simulink model "quadrotor_model50"  (R2021a)
settings: Solver=VariableStepAuto  StartTime=0.0  StopTime=40  RelTol=1e-1
values from neighbouring files (symbols this model uses):
  X = [X realx(index)]    [Plot_drone_3D.m]    (also in Plot_drone_3D_sub.m)
  Y = [Y realy(index)]    [Plot_drone_3D.m]    (also in Plot_drone_3D_sub.m)
  Z = [Z realz(index)]    [Plot_drone_3D.m]    (also in Plot_drone_3D_sub.m)
undefined symbols (not defined in the file or in its folder): Discrete, Time
libraries: sm_lib x6, sharedTrackingLibrary x4, sharedtransform x3, vrlib x2, aerolibutil x2, nesl_utility x1, dspmtrx3 x1, ctrlSharedLib x1
(part 1 of 2)
settings Model: EnablePacing=on  PacingRate=50  Creator=amejiyopakapak  LastModifiedBy=user
settings DataIOCC: ReturnWorkspaceOutputs=off
settings DebuggingCC: UnderSpecifiedDimensionMsg=warning

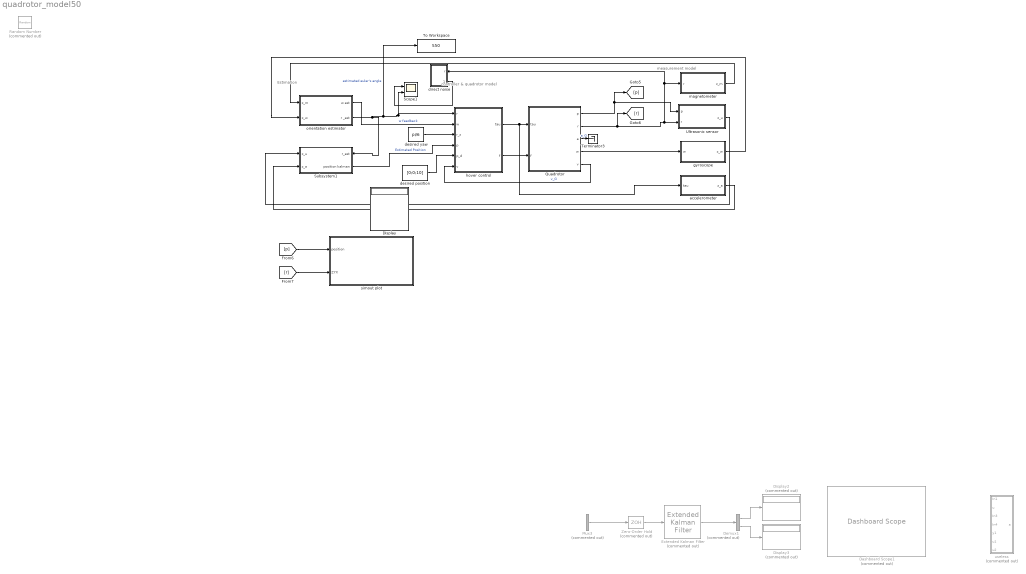
== system quadrotor_model50 ==
  note: Estimation
  note: measurement model
  note: controller & quadrotor model
  Dashboard Scope1 : DashboardScope  Commented=on
  Demux1 : Demux  Commented=on  Outputs=2
  Display : Display
  Display2 : Display  Commented=on
  Display3 : Display  Commented=on
  Extended Kalman Filter : sharedTrackingLibrary/Extended Kalman Filter  Commented=on  StateTransitionFcn=state  HasStateTransitionJacobianFcn=on  HasAdditiveProcessNoise=Nonadditive  ProcessNoise=[[1;1;1];[1;1;1]]  HasTimeVaryingProcessNoise=off  HasStateTransitionFcnExtraArgument=0  InitialState=[[0;0;0];[0;0;0]]  InitialStateCovariance=[[1;1;1];[1;1;1]]  MeasurementFcn1=measurement  HasMeasurementJacobianFcn1=off  HasMeasurementEnablePort1=off  HasAdditiveMeasurementNoise1=Additive  MeasurementNoise1=[[1;1;1];[1;1;1]]  HasTimeVaryingMeasurementNoise1=off  HasMeasurementFcnExtraArgument1=0  MeasurementFcn2=myMeasurementFcn  HasMeasurementJacobianFcn2=off  HasMeasurementEnablePort2=off  HasAdditiveMeasurementNoise2=Additive  MeasurementNoise2=1  HasTimeVaryingMeasurementNoise2=off  HasMeasurementFcnExtraArgument2=0  MeasurementFcn3=myMeasurementFcn  HasMeasurementJacobianFcn3=off  HasMeasurementEnablePort3=off  HasAdditiveMeasurementNoise3=Additive  MeasurementNoise3=1  HasTimeVaryingMeasurementNoise3=off  HasMeasurementFcnExtraArgument3=0  MeasurementFcn4=myMeasurementFcn  HasMeasurementJacobianFcn4=off  HasMeasurementEnablePort4=off  HasAdditiveMeasurementNoise4=Additive  MeasurementNoise4=1  HasTimeVaryingMeasurementNoise4=off  HasMeasurementFcnExtraArgument4=0  MeasurementFcn5=myMeasurementFcn  HasMeasurementJacobianFcn5=off  HasMeasurementEnablePort5=off  HasAdditiveMeasurementNoise5=Additive  MeasurementNoise5=1  HasTimeVaryingMeasurementNoise5=off  HasMeasurementFcnExtraArgument5=0  EnableMultirate=off  StateTransitionFcnSampleTime=1  MeasurementFcn1SampleTime=1  MeasurementFcn2SampleTime=1  MeasurementFcn3SampleTime=1  MeasurementFcn4SampleTime=1  MeasurementFcn5SampleTime=1  UseCurrentEstimator=on  OutputStateCovariance=off  DataType=double  SampleTime=0.01  NumberOfMeasurements=1
      settings: SourceProductBaseCode=CT,DR,TF,ID,LP,NV,AR,RO,RR,UV,VE
  Mux3 : Mux  Commented=on  Inputs=2
  Quadrotor : Subsystem
  Random Number : RandomNumber  Commented=on  SampleTime=0.1
  Scope1 : Scope  NumInputPorts=2
  Subsystem1 : Subsystem
      settings: PortSchema="{\"entries\":[{\"content\":{\"sides\":[{\"content\":{\"connectorIds\":[\"In1\",\"In2\"]},\"type\":\"ConnectorPlacement.EquallySpacedRectSide\",\"uuid\":\"ff0e47d5-67a6-410d-af15-00f9184d5f56\"},{\"content\":{\"connectorIds\":[\"In3\",\"Out1\"],\"side\":\"RIGHT\"},\"type\":\"ConnectorPlacement.EquallySpacedRectSide\",\"uuid\":\"3604025b-9f7e-46ce-b48f-09d2018bc808\"},{\"content\":{\"connectorIds\":[],\"side\":\"TOP\"},\"type\":\"ConnectorPlacement.EquallySpacedRectSide\",\"uuid\":\"c6ccdc8d-b714-489c-bc8f-943c64a4c150\"}]},\"type\":\"ConnectorPlacement.EquallySpacedConnector\",\"uuid\":\"6526fc3b-b978-451b-84c0-583e32a0b9e3\"}],\"packageUris\":[\"http://schema.mathworks.com/mf0/Connector/R2020b\"],\"version\":\"1.0\"}"
  Terminator3 : Terminator
  To Workspace : ToWorkspace  VariableName=S50  SaveFormat=Timeseries  SampleTime=1/50
  Ultrasonic sensor : Subsystem
  Zero-Order Hold : ZeroOrderHold  Commented=on  SampleTime=0.01
  accelerometer : Subsystem
  desired position : Constant  Value=[0;0;10]
  desired yaw : Constant  Value=pi/6
  direct noise : Subsystem
      settings: PortSchema="{\"entries\":[{\"content\":{\"sides\":[{\"content\":{\"connectorIds\":[]},\"type\":\"ConnectorPlacement.EquallySpacedRectSide\",\"uuid\":\"c51df378-8ff8-4d17-a243-2bd48f2a1343\"},{\"content\":{\"connectorIds\":[\"In1\",\"Out1\"],\"side\":\"RIGHT\"},\"type\":\"ConnectorPlacement.EquallySpacedRectSide\",\"uuid\":\"e335f112-6ed8-4a5c-b285-a63f6c692f38\"},{\"content\":{\"connectorIds\":[],\"side\":\"TOP\"},\"type\":\"ConnectorPlacement.EquallySpacedRectSide\",\"uuid\":\"f87c7cdc-99df-462c-be44-1c188cc81712\"}]},\"type\":\"ConnectorPlacement.EquallySpacedConnector\",\"uuid\":\"5aacd153-2f27-4b85-80cd-18cd67604917\"}],\"packageUris\":[\"http://schema.mathworks.com/mf0/Connector/R2020b\"],\"version\":\"1.0\"}"
  gyroscope : Subsystem
  hover control : Subsystem  mask{mass=1}
  magnetometer : Subsystem
      settings: PortSchema="{\"entries\":[{\"content\":{\"sides\":[{\"content\":{\"connectorIds\":[\"Out1\"]},\"type\":\"ConnectorPlacement.EquallySpacedRectSide\",\"uuid\":\"28b5311d-12b5-46a9-9a41-026d4bdaef13\"},{\"content\":{\"connectorIds\":[\"In1\"],\"side\":\"RIGHT\"},\"type\":\"ConnectorPlacement.EquallySpacedRectSide\",\"uuid\":\"3c807059-2a43-4a59-b0f2-7f82e794ec70\"},{\"content\":{\"connectorIds\":[],\"side\":\"TOP\"},\"type\":\"ConnectorPlacement.EquallySpacedRectSide\",\"uuid\":\"12203a37-ceaf-447f-ac57-ca6e6fe841d3\"}]},\"type\":\"ConnectorPlacement.EquallySpacedConnector\",\"uuid\":\"1f119634-8b2a-4a6d-a5af-b856cc81d6c9\"}],\"packageUris\":[\"http://schema.mathworks.com/mf0/Connector/R2020b\"],\"version\":\"1.0\"}"
  orientation estimator : Subsystem
  simout plot : Subsystem
  useless : Subsystem  Commented=on
  wires:
  desired yaw/1 -> hover control/3(r_z)
  Quadrotor/5(v) -> hover control/6(v)  "v_G"
  hover control/1(tau) -> accelerometer/1(tau), Quadrotor/1(tau)
  desired position/1 -> hover control/5(p_d)
  hover control/2(f) -> Quadrotor/2(f)
  Quadrotor/1(p) -> Ultrasonic sensor/1(p), [p]
  Mux3/1 -> Zero-Order Hold/1
  Extended Kalman Filter/1 -> Demux1/1
  Demux1/1 -> Display2/1
  Demux1/2 -> Display3/1
  Zero-Order Hold/1 -> Extended Kalman Filter/1
  orientation estimator/1(w est) -> hover control/2(w)  "w feedback"
  Quadrotor/4(w) -> gyroscope/1(w)
  Quadrotor/3(a) -> Terminator3/1  "a_G"
  magnetometer/1(z_m) -> orientation estimator/1(z_m)
  gyroscope/1(z_w) -> orientation estimator/2(z_w)
  accelerometer/1(z_a) -> Subsystem1/2(z_a)
  orientation estimator/2(r _est) -> Subsystem1/3(r_est), To Workspace/1, Scope1/2, hover control/1(r)  "estimated euler's angle"
  [p] -> simout plot/1(position)
  [r] -> simout plot/2(ZYX)
  Ultrasonic sensor/1(z_u) -> Subsystem1/1(z_u)
  Subsystem1/1(position kalman) -> hover control/4(p)  "Estimated Position"
  Quadrotor/2(r) -> direct noise/1(r), magnetometer/1(r), Ultrasonic sensor/2(r), [r]
  direct noise/1(ZYX) -> Scope1/1

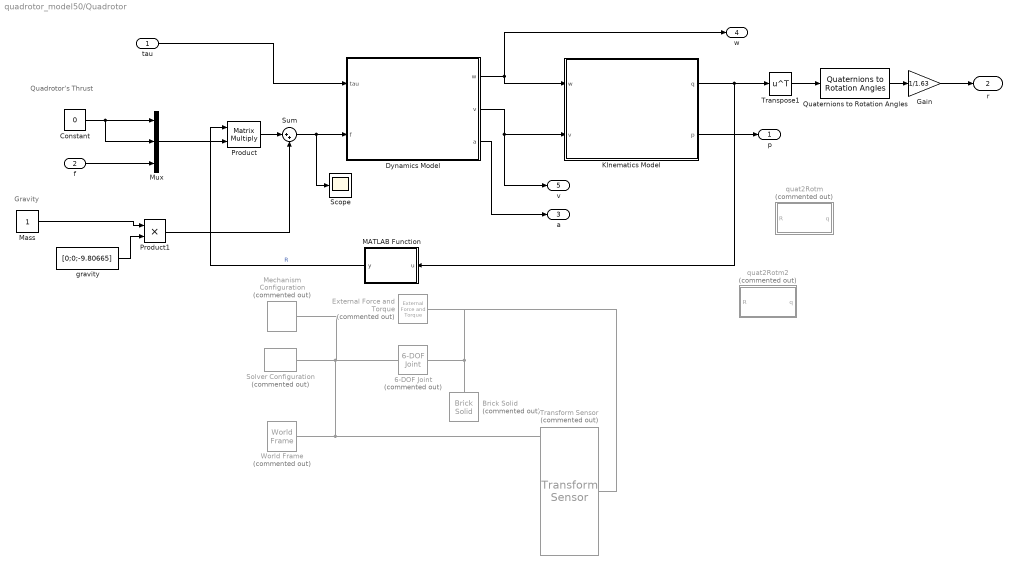
== system quadrotor_model50/Quadrotor ==
  note: Quadrotor's Thrust
  note: Gravity
  tau : Inport  SampleTime=1/50
  f : Inport  Port=2  SampleTime=1/50
  6-DOF Joint : sm_lib/Joints/6-DOF Joint  Commented=on  JointMode=Normal  SenseConstraintForce=off  SenseConstraintForceX=off  SenseConstraintForceY=off  SenseConstraintForceZ=off  SenseConstraintTorque=off  SenseConstraintTorqueX=off  SenseConstraintTorqueY=off  SenseConstraintTorqueZ=off  SenseTotalForce=off  SenseTotalForceX=off  SenseTotalForceY=off  SenseTotalForceZ=off  SenseTotalTorque=off  SenseTotalTorqueX=off  SenseTotalTorqueY=off  SenseTotalTorqueZ=off  CompositeWrenchDir=FollowerOnBase  CompositeWrenchFrame=BaseFrame  PxEquilibriumPosition=0  PxEquilibriumPositionUnits=m  PxSpringStiffness=0  PxSpringStiffnessUnits=N/m  PxDampingCoefficient=0  PxDampingCoefficientUnits=N/(m/s)  PxTorqueActuationMode=NoTorque  PxMotionActuationMode=ComputedMotion  PxSensePosition=off  PxSenseVelocity=off  PxSenseAcceleration=off  PxSenseTorqueForce=off  PxSenseLowerLimitTorqueForce=off  PxSenseUpperLimitTorqueForce=off  PxLowerLimitSpecify=off  PxLowerLimitBound=-1  PxLowerLimitBoundUnits=m  PxLowerLimitStiffness=1e6  PxLowerLimitStiffnessUnits=N/m  PxLowerLimitDamping=1e3  PxLowerLimitDampingUnits=N/(m/s)  PxLowerLimitTransitionRegionWidth=1e-4  PxLowerLimitTransitionRegionWidthUnits=m  PxUpperLimitSpecify=off  PxUpperLimitBound=1  PxUpperLimitBoundUnits=m  PxUpperLimitStiffness=1e6  PxUpperLimitStiffnessUnits=N/m  PxUpperLimitDamping=1e3  PxUpperLimitDampingUnits=N/(m/s)  PxUpperLimitTransitionRegionWidth=1e-4  PxUpperLimitTransitionRegionWidthUnits=m  PxPositionTargetSpecify=off  PxPositionTargetPriority=High  PxPositionTargetValue=0  PxPositionTargetValueUnits=m  PxVelocityTargetSpecify=off  PxVelocityTargetPriority=High  PxVelocityTargetValue=0  PxVelocityTargetValueUnits=m/s  PyEquilibriumPosition=0  PyEquilibriumPositionUnits=m  PySpringStiffness=0  PySpringStiffnessUnits=N/m  PyDampingCoefficient=0  PyDampingCoefficientUnits=N/(m/s)  PyTorqueActuationMode=NoTorque  PyMotionActuationMode=ComputedMotion  PySensePosition=off  PySenseVelocity=off  PySenseAcceleration=off  PySenseTorqueForce=off  PySenseLowerLimitTorqueForce=off  PySenseUpperLimitTorqueForce=off  PyLowerLimitSpecify=off  PyLowerLimitBound=-1  PyLowerLimitBoundUnits=m  PyLowerLimitStiffness=1e6  PyLowerLimitStiffnessUnits=N/m  PyLowerLimitDamping=1e3  PyLowerLimitDampingUnits=N/(m/s)  PyLowerLimitTransitionRegionWidth=1e-4  PyLowerLimitTransitionRegionWidthUnits=m  PyUpperLimitSpecify=off  PyUpperLimitBound=1  PyUpperLimitBoundUnits=m  PyUpperLimitStiffness=1e6  PyUpperLimitStiffnessUnits=N/m  PyUpperLimitDamping=1e3  PyUpperLimitDampingUnits=N/(m/s)  PyUpperLimitTransitionRegionWidth=1e-4  PyUpperLimitTransitionRegionWidthUnits=m  PyPositionTargetSpecify=off  PyPositionTargetPriority=High  PyPositionTargetValue=0  PyPositionTargetValueUnits=m  PyVelocityTargetSpecify=off  PyVelocityTargetPriority=High  PyVelocityTargetValue=0  PyVelocityTargetValueUnits=m/s  PzEquilibriumPosition=0  PzEquilibriumPositionUnits=m  PzSpringStiffness=0  PzSpringStiffnessUnits=N/m  PzDampingCoefficient=0  PzDampingCoefficientUnits=N/(m/s)  PzTorqueActuationMode=NoTorque  PzMotionActuationMode=ComputedMotion  PzSensePosition=off  PzSenseVelocity=off  PzSenseAcceleration=off  PzSenseTorqueForce=off  PzSenseLowerLimitTorqueForce=off  PzSenseUpperLimitTorqueForce=off  PzLowerLimitSpecify=off  PzLowerLimitBound=-1  PzLowerLimitBoundUnits=m  PzLowerLimitStiffness=1e6  PzLowerLimitStiffnessUnits=N/m  PzLowerLimitDamping=1e3  PzLowerLimitDampingUnits=N/(m/s)  PzLowerLimitTransitionRegionWidth=1e-4  PzLowerLimitTransitionRegionWidthUnits=m  PzUpperLimitSpecify=off  PzUpperLimitBound=1  PzUpperLimitBoundUnits=m  PzUpperLimitStiffness=1e6  PzUpperLimitStiffnessUnits=N/m  PzUpperLimitDamping=1e3  PzUpperLimitDampingUnits=N/(m/s)  PzUpperLimitTransitionRegionWidth=1e-4  PzUpperLimitTransitionRegionWidthUnits=m  PzPositionTargetSpecify=off  PzPositionTargetPriority=High  PzPositionTargetValue=0  PzPositionTargetValueUnits=m  PzVelocityTargetSpecify=off  PzVelocityTargetPriority=High  PzVelocityTargetValue=0  PzVelocityTargetValueUnits=m/s  SphDefPosRotationMethod=None  SphDefPosRotationAngleUnits=deg  SphDefPosRotationStandardAxis=+Z  SphDefPosRotationAngle=0.0  SphDefPosRotationArbitraryAxis=[0 0 1]  SphDefPosFollAlignAxisA=+X  SphDefPosBaseAlignAxisA=+Y  SphDefPosFollAlignAxisB=+Y  SphDefPosBaseAlignAxisB=+Z  SphDefPosRotationSequenceAxes=FollowerAxes  SphDefPosRotationSequence=XYX  SphDefPosRotationSequenceAngles=[0 0 0]  SphDefPosRotationSequenceAnglesUnits=deg  SphDefPosRotationMatrix=[1 0 0; 0 1 0; 0 0 1]  SphEqPosRotationMethod=None  SphEqPosRotationAngleUnits=deg  SphEqPosRotationStandardAxis=+Z  SphEqPosRotationAngle=0.0  SphEqPosRotationArbitraryAxis=[0 0 1]  SphEqPosFollAlignAxisA=+X  SphEqPosBaseAlignAxisA=+Y  SphEqPosFollAlignAxisB=+Y  SphEqPosBaseAlignAxisB=+Z  SphEqPosRotationSequenceAxes=FollowerAxes  SphEqPosRotationSequence=XYX  SphEqPosRotationSequenceAngles=[0 0 0]  SphEqPosRotationSequenceAnglesUnits=deg  SphEqPosRotationMatrix=[1 0 0; 0 1 0; 0 0 1]  SphSpringStiffness=0  SphSpringStiffnessUnits=N*m/deg  SphDampingCoefficient=0  SphDampingCoefficientUnits=N*m/(deg/s)  SphActuateTorqueX=off  SphActuateTorqueY=off  SphActuateTorqueZ=off  SphActuateTorque=off  SphTorqueActuationMode=NoTorque  SphMotionActuationMode=ComputedMotion  SphActuationFrame=BaseFrame  SphSensePosition=off  SphSenseVelocityX=off  SphSenseVelocityY=off  SphSenseVelocityZ=off  SphSenseVelocity=off  SphSenseAccelerationX=off  SphSenseAccelerationY=off  SphSenseAccelerationZ=off  SphSenseAcceleration=off  SphSenseTorqueX=off  SphSenseTorqueY=off  SphSenseTorqueZ=off  SphSenseTorqueForce=off  SphSenseLowerLimitTorqueMag=off  SphSenseUpperLimitTorqueMag=off  SphSensingFrame=BaseFrame  SphLowerLimitSpecify=off  SphLowerLimitBound=15  SphLowerLimitBoundUnits=deg  SphLowerLimitStiffness=1e4  SphLowerLimitStiffnessUnits=N*m/deg  SphLowerLimitDamping=10  SphLowerLimitDampingUnits=N*m/(deg/s)  SphLowerLimitTransitionRegionWidth=0.1  SphLowerLimitTransitionRegionWidthUnits=deg  SphUpperLimitSpecify=off  SphUpperLimitBound=45  SphUpperLimitBoundUnits=deg  SphUpperLimitStiffness=1e4  SphUpperLimitStiffnessUnits=N*m/deg  SphUpperLimitDamping=10  SphUpperLimitDampingUnits=N*m/(deg/s)  SphUpperLimitTransitionRegionWidth=0.1  SphUpperLimitTransitionRegionWidthUnits=deg  SphPositionTargetRotationMethod=None  SphPositionTargetRotationAngleUnits=deg  SphPositionTargetRotationStandardAxis=+Z  SphPositionTargetRotationAngle=0.0  SphPositionTargetRotationArbitraryAxis=[0 0 1]  SphPositionTargetFollAlignAxisA=+X  SphPositionTargetBaseAlignAxisA=+Y  SphPositionTargetFollAlignAxisB=+Y  SphPositionTargetBaseAlignAxisB=+Z  SphPositionTargetRotationSequenceAxes=FollowerAxes  SphPositionTargetRotationSequence=XYX  SphPositionTargetRotationSequenceAngles=[0 0 0]  SphPositionTargetRotationSequenceAnglesUnits=deg  SphPositionTargetRotationMatrix=[1 0 0; 0 1 0; 0 0 1]  SphPositionTargetSpecify=off  SphPositionTargetPriority=High  SphVelocityTargetValue=[0 0 0]  SphVelocityTargetValueUnits=deg/s  SphVelocityTargetSpecify=off  SphVelocityTargetPriority=High  SphVelocityTargetInFollowerFrame=on
  Brick Solid : sm_lib/Body Elements/Brick Solid  Commented=on  GraphicAmbientColor=[0.15 0.15 0.15 1.0]  BasedOnType=Density  BrickDimensions=[1 1 1]  BrickDimensionUnits=m  CenterOfMass=[0 0 0]  CenterOfMassUnits=m  GraphicDiffuseColor=[0.5 0.5 0.5]  Density=1000  DensityUnits=kg/m^3  DoExposeReferenceFrame=on  GraphicEmissiveColor=[0.0 0.0 0.0 1.0]  ExportEntireGeometry=off  SerializedFrames=<Frames/>  MarkerShape=Sphere  MarkerSize=10  GraphicType=FromGeometry  InertiaType=CalculateFromGeometry  Mass=1  MassUnits=kg  MomentsOfInertia=[1 1 1]  MomentsOfInertiaUnits=kg*m^2  GraphicOpacity=1.0  ProductsOfInertia=[0 0 0]  ProductsOfInertiaUnits=kg*m^2  GraphicShininess=75  GraphicSpecularColor=[0.5 0.5 0.5 1.0]  GraphicVisPropType=SimpleVisualProperties
  Constant : Constant  Value=0
  Dynamics Model : Subsystem  mask{I=[1 0 0 ; 0 1 0; 0 0 1], m=1, w_0=[0;0;0], v_0=[0;0;0]}
      mask prompts: I "Body Inertia Matrix"; m "Mass"; w_0 "Initial Angular Velocity"; v_0 "Initial Linear Velocity"
      mask DialogControl Container3 Prompt: Physical Parameters
      mask DialogControl Container4 Prompt: Initial States
      mask Display: disp('Dynamics Model')
  External Force and Torque : sm_lib/Forces and Torques/External Force and Torque  Commented=on  ForceResolutionFrame=AttachedFrame  EnableForceX=off  EnableForceY=off  EnableForceZ=off  EnableForce=on  TorqueResolutionFrame=AttachedFrame  EnableTorqueX=off  EnableTorqueY=off  EnableTorqueZ=off  EnableTorque=on
  Gain : Gain  Gain=1/1.63
  "KInematics Model " : Subsystem  mask{q_0=[1;0;0;0], p_0=[0;0;0]}
      mask prompts: q_0 "Initial Orienetation (in quaternion)"; p_0 "Initial Position"
      mask DialogControl Container3 Prompt: Initial States
      mask Display: disp('Kinematics Model')
  MATLAB Function : MATLAB Function  TreatAsAtomicUnit=on
  Mass : Constant
  Mechanism Configuration : sm_lib/Utilities/Mechanism Configuration  Commented=on  UniformGravity=Constant  GravityVector=[0 0 -9.80665]  GravityVectorUnits=m/s^2  GravityUnits=m/s^2  LinearizationDelta=0.001  JointModeTransitionNonlinearIterations=2
  Mux : Mux  Inputs=3
  Product : Product  Multiplication=Matrix(*)
  Product1 : Product
  Quaternions to Rotation Angles : sharedtransform/Quaternions to Rotation Angles  rotationOrder=ZYX  aMode=aMode
      settings: SourceProductBaseCode=AE,PW,DR,MT,UV,VE
  Scope : Scope
  Solver Configuration : nesl_utility/Solver Configuration  Commented=on  PhysicalDomain=network_engine_domain  SubClassName=solver  LeftPortType=input  RightPortType=generic  Tones=[]  Harmonics=[]  SimulateNoise=off  Profile=off  UseLocalSampling=off  EnableSwitchedLinearOptims=on  FrequencyDomain=off  UseCCode=off  RelTol=0.001  AbsTol=1e-06  MinStep=1e-09  ToWorkspace=off  RevertToSquareIcSolve=off  NumHomotopyIterations=100  PhasorMode=off  PhasorModeNumHarmonics=1  DoDC=off  ResidualTolerance=1e-09  UseLocalSolver=off  LocalSolverChoice=NE_BACKWARD_EULER_ADVANCER  LocalSolverSampleTime=0.001  DoFixedCost=off  MaxNonlinIter=3  MaxModeIter=2  ComputeImpulses=off  ImpulseIterations=2  LinearAlgebra=auto  EquationFormulation=NE_TIME_EF  DelaysMemoryBudget=1024  AutomaticFiltering=on  FilteringTimeConstant=0.001  PartitionStorageMethod=AS_NEEDED  PartitionMemoryBudget=1024  PartitionMethod=ROBUST
  Sum : Sum  Inputs=|++
  Transform Sensor : sm_lib/Frames and Transforms/Transform Sensor  Commented=on  MeasurementFrame=World  SenseAngle=off  SenseAxis=off  SenseAngle1=off  SenseAngle2=off  SenseAngle3=off  SenseQ=on  SenseR=off  SenseOmegaX=on  SenseOmegaY=on  SenseOmegaZ=on  SenseOmega1=off  SenseOmega2=off  SenseOmega3=off  SenseQDot=off  SenseRDot=off  SenseAlphaX=off  SenseAlphaY=off  SenseAlphaZ=off  SenseAlpha1=off  SenseAlpha2=off  SenseAlpha3=off  SenseQDDot=off  SenseRDDot=off  SenseX=on  SenseY=on  SenseZ=on  SenseRad=off  SenseAzim=off  SenseDist=off  SenseInc=off  SenseXDot=on  SenseYDot=on  SenseZDot=on  SenseRadDot=off  SenseAzimDot=off  SenseDistDot=off  SenseIncDot=off  SenseXDDot=off  SenseYDDot=off  SenseZDDot=off  SenseRadDDot=off  SenseAzimDDot=off  SenseDistDDot=off  SenseIncDDot=off
  Transpose1 : Math  Operator=transpose  SaturateOnIntegerOverflow=on
  World Frame : sm_lib/Frames and Transforms/World Frame  Commented=on
  gravity : Constant  Value=[0;0;-9.80665]
  quat2Rotm : Subsystem  Commented=on
      mask Display: disp('R(q)')
  quat2Rotm2 : Subsystem  Commented=on
      mask Display: disp('R(q)')
  p : Outport  SampleTime=1/50
  r : Outport  Port=2  SampleTime=1/50
  a : Outport  Port=3  SampleTime=1/50
  w : Outport  Port=4  SampleTime=1/50
  v : Outport  Port=5  SampleTime=1/50
  wires:
  Dynamics Model/1(w) -> "KInematics Model "/1(w), w/1
  "KInematics Model "/2(p) -> p/1
  Dynamics Model/2(v) -> v/1, "KInematics Model "/2(v)
  f/1 -> Mux/3
  Constant/1 -> Mux/2, Mux/1
  Product/1 -> Sum/1
  Product1/1 -> Sum/2
  gravity/1 -> Product1/2
  Mass/1 -> Product1/1
  Dynamics Model/3(a) -> a/1
  MATLAB Function/1(y) -> Product/1  "R"
  Mux/1 -> Product/2
  Sum/1 -> Scope/1, Dynamics Model/2(f)
  tau/1 -> Dynamics Model/1(tau)
  "KInematics Model "/1(q) -> Transpose1/1, MATLAB Function/1(u)
  Transpose1/1 -> Quaternions to Rotation Angles/1
  Quaternions to Rotation Angles/1 -> Gain/1
  Gain/1 -> r/1
  connections:
  Solver Configuration/RConn1 -- Mechanism Configuration/RConn1 -- 6-DOF Joint/LConn1 -- Transform Sensor/RConn1 -- World Frame/RConn1
  6-DOF Joint/RConn1 -- External Force and Torque/RConn1 -- Transform Sensor/LConn1 -- Brick Solid/RConn1

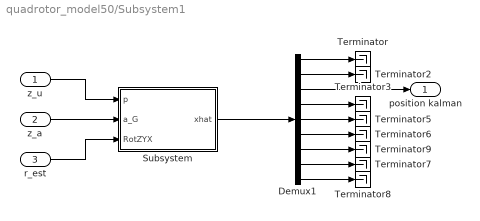
== system quadrotor_model50/Subsystem1 ==
  z_u : Inport
  z_a : Inport  Port=2
  r_est : Inport  Port=3
  Demux1 : Demux  Outputs=9
  Subsystem : Subsystem
  Terminator{,2..3,5..9} (8 alike) : Terminator
  position kalman : Outport
  wires:
  Demux1/5 -> Terminator5/1
  Demux1/1 -> Terminator/1
  Demux1/8 -> Terminator7/1
  Demux1/4 -> Terminator3/1
  Demux1/9 -> Terminator8/1
  Demux1/6 -> Terminator6/1
  Demux1/7 -> Terminator9/1
  Demux1/2 -> Terminator2/1
  r_est/1 -> Subsystem/3(RotZYX)
  Subsystem/1(xhat) -> Demux1/1
  Demux1/3 -> position kalman/1
  z_u/1 -> Subsystem/1(p)
  z_a/1 -> Subsystem/2(a_G)

== system quadrotor_model50/Ultrasonic sensor ==
  p : Inport
  r : Inport  Port=2
  Demux : Demux  Outputs=3
  Divide : Product  Inputs=*/
  MATLAB Function : MATLAB Function  TreatAsAtomicUnit=on
  Random Number1 : RandomNumber  Variance=0.05  SampleTime=0.05
  Sum : Sum  Inputs=|++
  Terminator : Terminator
  z_u : Outport
  wires:
  r/1 -> Demux/1
  Demux/1 -> Terminator/1
  Demux/2 -> MATLAB Function/1(u1)
  Demux/3 -> MATLAB Function/2(u2)
  p/1 -> Divide/1
  MATLAB Function/1(y) -> Divide/2
  Sum/1 -> z_u/1
  Divide/1 -> Sum/1
  Random Number1/1 -> Sum/2

== system quadrotor_model50/accelerometer ==
  tau : Inport
  Demux3 : Demux  Outputs=3
  Divide : Product  Inputs=*/
  Mux1 : Mux  Inputs=3
  Random Number2 : RandomNumber  Variance=0.000001  SampleTime=0.01
  Sum1 : Sum  Inputs=|++
  mass : Constant
  z_a : Outport
  wires:
  tau/1 -> Divide/1
  Demux3/2 -> Mux1/2
  mass/1 -> Divide/2
  Random Number2/1 -> Sum1/2
  Demux3/3 -> Sum1/1
  Divide/1 -> Demux3/1
  Mux1/1 -> z_a/1
  Demux3/1 -> Mux1/1
  Sum1/1 -> Mux1/3

== system quadrotor_model50/direct noise ==
  r : Inport
  Demux : Demux  Outputs=3
  Mux : Mux  Inputs=3
  Random Number2 : RandomNumber  Variance=0.001  SampleTime=0.01
  Sum1 : Sum  Inputs=|++
  ZYX : Outport
  wires:
  Random Number2/1 -> Sum1/1
  r/1 -> Demux/1
  Demux/1 -> Sum1/2
  Sum1/1 -> Mux/1
  Demux/2 -> Mux/2
  Demux/3 -> Mux/3
  Mux/1 -> ZYX/1

== system quadrotor_model50/gyroscope ==
  w : Inport
  Demux3 : Demux  Outputs=3
  Mux1 : Mux  Inputs=3
  Random Number2 : RandomNumber  Variance=0.00005  SampleTime=0.03
  Sum1 : Sum  Inputs=|++
  z_w : Outport
  wires:
  Mux1/1 -> z_w/1
  Demux3/3 -> Sum1/1
  Random Number2/1 -> Sum1/2
  Sum1/1 -> Mux1/3
  Demux3/2 -> Mux1/2
  Demux3/1 -> Mux1/1
  w/1 -> Demux3/1

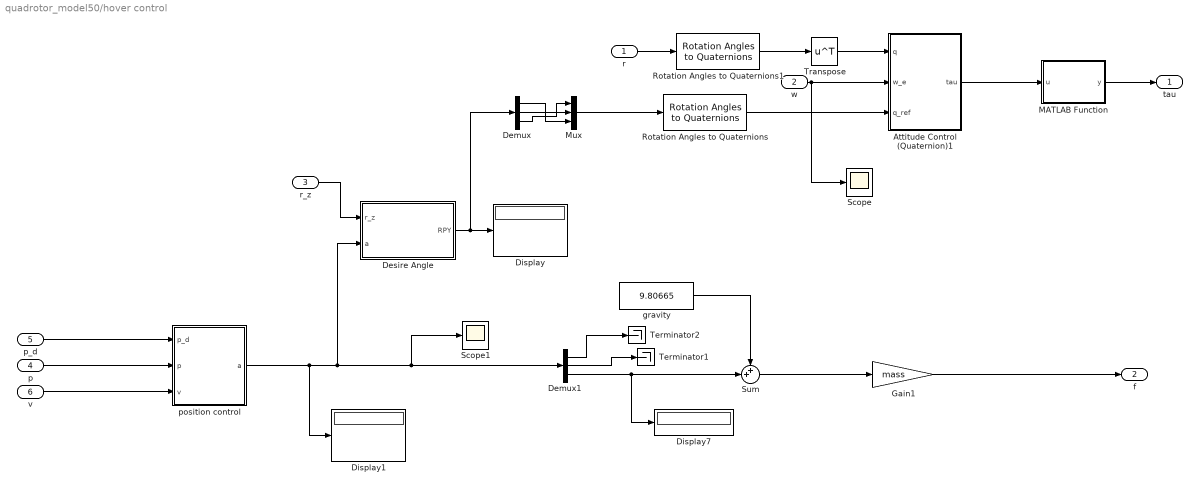
== system quadrotor_model50/hover control ==
  r : Inport  SampleTime=1/50
  w : Inport  Port=2
  r_z : Inport  Port=3  SampleTime=1/50
  p : Inport  Port=4  SampleTime=1/50
  p_d : Inport  Port=5  SampleTime=1/100
  v : Inport  Port=6  SampleTime=1/50
  Attitude Control (Quaternion)1 : Subsystem  mask{K_q=1.87426*diag([1;1;1]), K_w=8.1652*diag([1;1;1])}
      mask prompts: K_q "Proportional Gain"; K_w "Velocity Gain"
      mask DialogControl Container3 Prompt: Control Gain
  Demux : Demux  Outputs=3
  Demux1 : Demux  Outputs=3
  Desire Angle : Subsystem
  Display : Display
  Display1 : Display
  Display7 : Display
  Gain1 : Gain  Gain=mass
  MATLAB Function : MATLAB Function  TreatAsAtomicUnit=on
  Mux : Mux  Inputs=3
  Rotation Angles to Quaternions : sharedtransform/Rotation Angles to Quaternions  rotationOrder=ZYX  aMode=aMode
      settings: SourceProductBaseCode=AE,PW,DR,MT,UV,VE
  Rotation Angles to Quaternions1 : sharedtransform/Rotation Angles to Quaternions  rotationOrder=ZYX  aMode=aMode
      settings: SourceProductBaseCode=AE,PW,DR,MT,UV,VE
  Scope : Scope
  Scope1 : Scope
  Sum : Sum  Inputs=++|
  Terminator1 : Terminator
  Terminator2 : Terminator
  Transpose : Math  Operator=transpose  SaturateOnIntegerOverflow=on
  gravity : Constant  Value=9.80665  VectorParams1D=off
  position control : Subsystem  mask{K_p=2.2*diag([0;0;1]), K_d=1.5*diag([0;0;1]), K_i=0*diag([1;1;1])}
  tau : Outport  SampleTime=1/50
  f : Outport  Port=2  SampleTime=1/50
  wires:
  Rotation Angles to Quaternions/1 -> Attitude Control (Quaternion)1/3(q_ref)
  Demux1/2 -> Terminator1/1
  Sum/1 -> Gain1/1
  Demux1/3 -> Display7/1, Sum/2
  MATLAB Function/1(y) -> tau/1
  Attitude Control (Quaternion)1/1(tau) -> MATLAB Function/1(u)
  gravity/1 -> Sum/1
  Demux1/1 -> Terminator2/1
  Mux/1 -> Rotation Angles to Quaternions/1
  w/1 -> Attitude Control (Quaternion)1/2(w_e), Scope/1
  v/1 -> position control/3(v)
  r_z/1 -> Desire Angle/1(r_z)
  p_d/1 -> position control/1(p_d)
  p/1 -> position control/2(p)
  position control/1(a) -> Scope1/1, Demux1/1, Desire Angle/2(a), Display1/1
  Gain1/1 -> f/1
  Demux/2 -> Mux/2
  Demux/1 -> Mux/3
  Demux/3 -> Mux/1
  Desire Angle/1(RPY) -> Demux/1, Display/1
  Rotation Angles to Quaternions1/1 -> Transpose/1
  r/1 -> Rotation Angles to Quaternions1/1
  Transpose/1 -> Attitude Control (Quaternion)1/1(q)

== system quadrotor_model50/magnetometer ==
  r : Inport  SampleTime=1/100
  Constant2 : Constant  Value=0  SampleTime=1/100
  Demux : Demux  Outputs=3
  MATLAB Function : MATLAB Function  TreatAsAtomicUnit=on
  Mux : Mux  Inputs=3
  Mux1 : Mux  Inputs=3
  Product : Product  Multiplication=Matrix(*)
  Random Number2 : RandomNumber  Variance=0.000001  SampleTime=0.01
  Sum1 : Sum  Inputs=|++
  north magnetic : Constant  SampleTime=1/100
  z_m : Outport  SampleTime=1/100
  wires:
  MATLAB Function/1(y) -> Product/1
  r/1 -> Demux/1
  north magnetic/1 -> Mux1/2
  Constant2/1 -> Mux1/3, Mux1/1
  Mux1/1 -> Product/2
  Mux/1 -> MATLAB Function/1(u)
  Demux/2 -> Mux/2
  Demux/1 -> Mux/3
  Demux/3 -> Mux/1
  Product/1 -> Sum1/1
  Sum1/1 -> z_m/1
  Random Number2/1 -> Sum1/2

== system quadrotor_model50/orientation estimator ==
  z_m : Inport  SampleTime=1/50
  z_w : Inport  Port=2  SampleTime=1/50
  Demux : Demux  Outputs=9
  Extended Kalman Filter : sharedTrackingLibrary/Extended Kalman Filter  StateTransitionFcn=myStateTransitionFcn  HasStateTransitionJacobianFcn=on  StateTransitionJacobianFcn=jacoState  HasAdditiveProcessNoise=Nonadditive  ProcessNoise=diag([0;0;0;0;0;0;0;0;0])  HasTimeVaryingProcessNoise=off  HasStateTransitionFcnExtraArgument=0  InitialState=[0;0;0;0;0;0;0;0;0]  InitialStateCovariance=diag([1e-1;1e-1;0.5;1e-9;1e-9;1e-7;1e-20;1e-20;1e-5])  MeasurementFcn1=myMeasurementFcn  HasMeasurementJacobianFcn1=on  MeasurementJacobianFcn1=jacomeasure  HasMeasurementEnablePort1=off  HasAdditiveMeasurementNoise1=Additive  MeasurementNoise1=diag([1e-12;1e-12;1.4e-3;3;3;0.001])  HasTimeVaryingMeasurementNoise1=off  HasMeasurementFcnExtraArgument1=0  MeasurementFcn2=myMeasurementFcnOmega  HasMeasurementJacobianFcn2=off  HasMeasurementEnablePort2=off  HasAdditiveMeasurementNoise2=Additive  MeasurementNoise2=1  HasTimeVaryingMeasurementNoise2=off  HasMeasurementFcnExtraArgument2=0  MeasurementFcn3=myMeasurementFcn  HasMeasurementJacobianFcn3=off  HasMeasurementEnablePort3=off  HasAdditiveMeasurementNoise3=Additive  MeasurementNoise3=1  HasTimeVaryingMeasurementNoise3=off  HasMeasurementFcnExtraArgument3=0  MeasurementFcn4=myMeasurementFcn  HasMeasurementJacobianFcn4=off  HasMeasurementEnablePort4=off  HasAdditiveMeasurementNoise4=Additive  MeasurementNoise4=1  HasTimeVaryingMeasurementNoise4=off  HasMeasurementFcnExtraArgument4=0  MeasurementFcn5=myMeasurementFcn  HasMeasurementJacobianFcn5=off  HasMeasurementEnablePort5=off  HasAdditiveMeasurementNoise5=Additive  MeasurementNoise5=1  HasTimeVaryingMeasurementNoise5=off  HasMeasurementFcnExtraArgument5=0  EnableMultirate=off  StateTransitionFcnSampleTime=1/100  MeasurementFcn1SampleTime=1/100  MeasurementFcn2SampleTime=1  MeasurementFcn3SampleTime=1  MeasurementFcn4SampleTime=1  MeasurementFcn5SampleTime=1  UseCurrentEstimator=on  OutputStateCovariance=off  DataType=double  SampleTime=1/50  NumberOfMeasurements=1
      settings: SourceProductBaseCode=CT,DR,TF,ID,LP,NV,AR,RO,RR,UV,VE
  Mux : Mux  Inputs=2
  Mux1 : Mux  Inputs=3
  Mux2 : Mux  Inputs=3
  Terminator : Terminator
  Terminator1 : Terminator
  Terminator2 : Terminator
  Zero-Order Hold : ZeroOrderHold  SampleTime=1/50
  w est : Outport  SampleTime=1/50
  r _est : Outport  Port=2  SampleTime=1/50
  wires:
  Extended Kalman Filter/1 -> Demux/1
  Zero-Order Hold/1 -> Extended Kalman Filter/1
  Mux/1 -> Zero-Order Hold/1
  Demux/1 -> Mux1/1
  z_m/1 -> Mux/2
  Demux/7 -> Mux2/3
  Demux/2 -> Mux1/2
  Demux/9 -> Mux2/1
  Demux/8 -> Mux2/2
  Mux1/1 -> w est/1
  z_w/1 -> Mux/1
  Demux/3 -> Mux1/3
  Demux/4 -> Terminator/1
  Demux/5 -> Terminator1/1
  Demux/6 -> Terminator2/1
  Mux2/1 -> r _est/1

== system quadrotor_model50/simout plot ==
  position : Inport
  ZYX : Inport  Port=2
  Clock : Clock
  To Workspace : ToWorkspace  VariableName=ZYX  SampleTime=0.05
      settings: Save2DSignal=2-D array (concatenate along first dimension)
  To Workspace1 : ToWorkspace  VariableName=position  SampleTime=0.05
  To Workspace2 : ToWorkspace  VariableName=time  SampleTime=0.05
      settings: Save2DSignal=2-D array (concatenate along first dimension)
  wires:
  ZYX/1 -> To Workspace/1
  position/1 -> To Workspace1/1
  Clock/1 -> To Workspace2/1

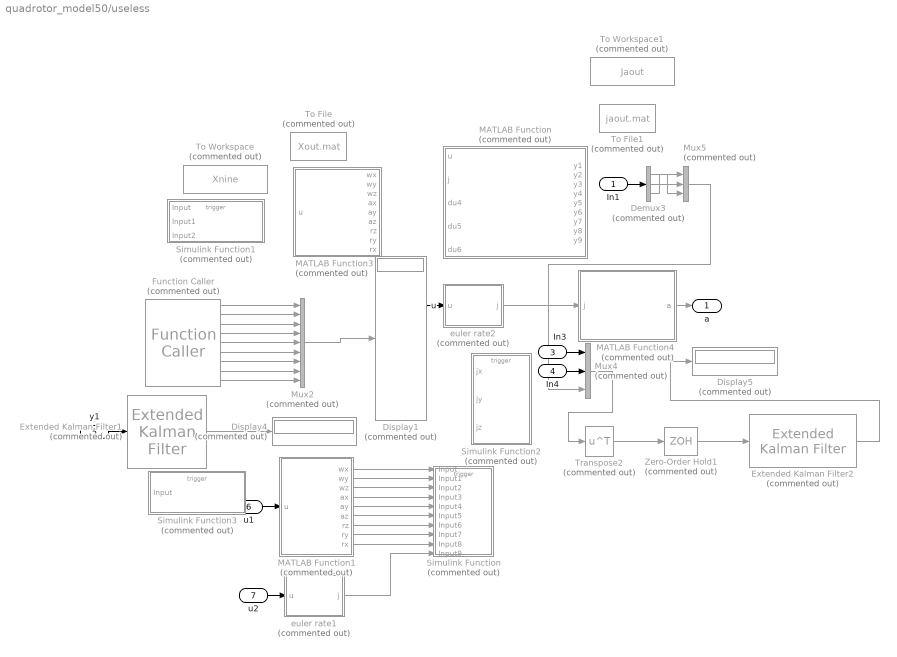
== system quadrotor_model50/useless ==
  In1 : Inport
  u : Inport  Port=2
  In3 : Inport  Port=3
  In4 : Inport  Port=4
  y1 : Inport  Port=5
  u1 : Inport  Port=6
  u2 : Inport  Port=7
  Demux3 : Demux  Commented=on  Outputs=3
  Display1 : Display  Commented=on
  Display4 : Display  Commented=on
  Display5 : Display  Commented=on
  Extended Kalman Filter1 : sharedTrackingLibrary/Extended Kalman Filter  Commented=on  StateTransitionFcn=suktee  HasStateTransitionJacobianFcn=on  StateTransitionJacobianFcn=jaba  HasAdditiveProcessNoise=Nonadditive  ProcessNoise=[1]  HasTimeVaryingProcessNoise=off  HasStateTransitionFcnExtraArgument=0  InitialState=[0;0;0;0;0;0;0;0;0]  InitialStateCovariance=[1;1;1;1;1;1;1;1;1]  MeasurementFcn1=messi  HasMeasurementJacobianFcn1=off  HasMeasurementEnablePort1=off  HasAdditiveMeasurementNoise1=Additive  MeasurementNoise1=[1;1;1]  HasTimeVaryingMeasurementNoise1=off  HasMeasurementFcnExtraArgument1=0  MeasurementFcn2=myMeasurementFcn  HasMeasurementJacobianFcn2=off  HasMeasurementEnablePort2=off  HasAdditiveMeasurementNoise2=Additive  MeasurementNoise2=1  HasTimeVaryingMeasurementNoise2=off  HasMeasurementFcnExtraArgument2=0  MeasurementFcn3=myMeasurementFcn  HasMeasurementJacobianFcn3=off  HasMeasurementEnablePort3=off  HasAdditiveMeasurementNoise3=Additive  MeasurementNoise3=1  HasTimeVaryingMeasurementNoise3=off  HasMeasurementFcnExtraArgument3=0  MeasurementFcn4=myMeasurementFcn  HasMeasurementJacobianFcn4=off  HasMeasurementEnablePort4=off  HasAdditiveMeasurementNoise4=Additive  MeasurementNoise4=1  HasTimeVaryingMeasurementNoise4=off  HasMeasurementFcnExtraArgument4=0  MeasurementFcn5=myMeasurementFcn  HasMeasurementJacobianFcn5=off  HasMeasurementEnablePort5=off  HasAdditiveMeasurementNoise5=Additive  MeasurementNoise5=1  HasTimeVaryingMeasurementNoise5=off  HasMeasurementFcnExtraArgument5=0  EnableMultirate=off  StateTransitionFcnSampleTime=1  MeasurementFcn1SampleTime=1  MeasurementFcn2SampleTime=1  MeasurementFcn3SampleTime=1  MeasurementFcn4SampleTime=1  MeasurementFcn5SampleTime=1  UseCurrentEstimator=off  OutputStateCovariance=off  DataType=double  SampleTime=1  NumberOfMeasurements=1
      settings: SourceProductBaseCode=CT,DR,TF,ID,LP,NV,AR,RO,RR,UV,VE
  Extended Kalman Filter2 : sharedTrackingLibrary/Extended Kalman Filter  Commented=on  StateTransitionFcn=myStateTransitionFcnlong  HasStateTransitionJacobianFcn=on  StateTransitionJacobianFcn=jacolong  HasAdditiveProcessNoise=Nonadditive  ProcessNoise=[1; 1; 1; 1; 1; 1; 1; 1; 1]  HasTimeVaryingProcessNoise=off  HasStateTransitionFcnExtraArgument=0  InitialState=[0;0;0;0;0;0;0;0;0]  InitialStateCovariance=[1; 1; 1; 1; 1; 1; 1; 1; 1]  MeasurementFcn1=myMeasurementFcnlong  HasMeasurementJacobianFcn1=off  HasMeasurementEnablePort1=off  HasAdditiveMeasurementNoise1=Additive  MeasurementNoise1=[1; 1; 1;]  HasTimeVaryingMeasurementNoise1=off  HasMeasurementFcnExtraArgument1=0  MeasurementFcn2=myMeasurementFcn  HasMeasurementJacobianFcn2=off  HasMeasurementEnablePort2=off  HasAdditiveMeasurementNoise2=Additive  MeasurementNoise2=1  HasTimeVaryingMeasurementNoise2=off  HasMeasurementFcnExtraArgument2=0  MeasurementFcn3=myMeasurementFcn  HasMeasurementJacobianFcn3=off  HasMeasurementEnablePort3=off  HasAdditiveMeasurementNoise3=Additive  MeasurementNoise3=1  HasTimeVaryingMeasurementNoise3=off  HasMeasurementFcnExtraArgument3=0  MeasurementFcn4=myMeasurementFcn  HasMeasurementJacobianFcn4=off  HasMeasurementEnablePort4=off  HasAdditiveMeasurementNoise4=Additive  MeasurementNoise4=1  HasTimeVaryingMeasurementNoise4=off  HasMeasurementFcnExtraArgument4=0  MeasurementFcn5=myMeasurementFcn  HasMeasurementJacobianFcn5=off  HasMeasurementEnablePort5=off  HasAdditiveMeasurementNoise5=Additive  MeasurementNoise5=1  HasTimeVaryingMeasurementNoise5=off  HasMeasurementFcnExtraArgument5=0  EnableMultirate=on  StateTransitionFcnSampleTime=9  MeasurementFcn1SampleTime=3  MeasurementFcn2SampleTime=1  MeasurementFcn3SampleTime=1  MeasurementFcn4SampleTime=1  MeasurementFcn5SampleTime=1  UseCurrentEstimator=on  OutputStateCovariance=off  DataType=double  SampleTime=1/100  NumberOfMeasurements=1
      settings: SourceProductBaseCode=CT,DR,TF,ID,LP,NV,AR,RO,RR,UV,VE
  Function Caller : FunctionCaller  Commented=on  FunctionPrototype=[y1,y2,y3,y4,y5,y6,y7,y8,y9] = f()  InputArgumentSpecifications=<Enter example>  OutputArgumentSpecifications=<Enter example>
  MATLAB Function : MATLAB Function  Commented=on  TreatAsAtomicUnit=on
  MATLAB Function1 : MATLAB Function  Commented=on  TreatAsAtomicUnit=on
  MATLAB Function3 : MATLAB Function  Commented=on  TreatAsAtomicUnit=on
  MATLAB Function4 : MATLAB Function  Commented=on  TreatAsAtomicUnit=on
  Mux2 : Mux  Commented=on  Inputs=9
  Mux4 : Mux  Commented=on  Inputs=3
  Mux5 : Mux  Commented=on  Inputs=3
  Simulink Function : Subsystem  Commented=on  TreatAsAtomicUnit=on
  Simulink Function1 : Subsystem  Commented=on  TreatAsAtomicUnit=on
  Simulink Function2 : Subsystem  Commented=on  TreatAsAtomicUnit=on
  Simulink Function3 : Subsystem  Commented=on  TreatAsAtomicUnit=on
  To File : ToFile  Commented=on  Filename=Xout.mat  MatrixName=Xout  SaveFormat=Timeseries
  To File1 : ToFile  Commented=on  Filename=jaout.mat  MatrixName=jaout  SaveFormat=Timeseries
  To Workspace : ToWorkspace  Commented=on  VariableName=Xnine  SaveFormat=Timeseries  SampleTime=-1
  To Workspace1 : ToWorkspace  Commented=on  VariableName=Jaout  SaveFormat=Timeseries  SampleTime=-1
  Transpose2 : Math  Commented=on  Operator=transpose  SaturateOnIntegerOverflow=on
  Zero-Order Hold1 : ZeroOrderHold  Commented=on  SampleTime=0.01
  euler rate1 : MATLAB Function  Commented=on  TreatAsAtomicUnit=on
  euler rate2 : MATLAB Function  Commented=on  TreatAsAtomicUnit=on
  a : Outport
  wires:
  MATLAB Function1/8(ry) -> Simulink Function/8(Input7)
  Function Caller/3 -> Mux2/3
  Function Caller/9 -> Mux2/9
  u/1 -> euler rate2/1(u)
  Mux2/1 -> Display1/1
  Function Caller/1 -> Mux2/1
  MATLAB Function1/2(wy) -> Simulink Function/2(Input1)
  MATLAB Function4/1(a) -> a/1
  MATLAB Function1/6(az) -> Simulink Function/6(Input5)
  MATLAB Function1/5(ay) -> Simulink Function/5(Input4)
  MATLAB Function1/4(ax) -> Simulink Function/4(Input3)
  MATLAB Function1/7(rz) -> Simulink Function/7(Input6)
  Function Caller/4 -> Mux2/4
  u1/1 -> MATLAB Function1/1(u)
  Function Caller/5 -> Mux2/5
  Function Caller/2 -> Mux2/2
  Function Caller/6 -> Mux2/6
  Mux4/1 -> Transpose2/1
  MATLAB Function1/9(rx) -> Simulink Function/9(Input8)
  Demux3/2 -> Mux5/2
  Function Caller/7 -> Mux2/7
  MATLAB Function1/1(wx) -> Simulink Function/1(Input)
  Mux5/1 -> Mux4/3
  In4/1 -> Mux4/2
  u2/1 -> euler rate1/1(u)
  Zero-Order Hold1/1 -> Extended Kalman Filter2/1
  Extended Kalman Filter1/1 -> Display4/1
  Demux3/3 -> Mux5/1
  Extended Kalman Filter2/1 -> Display5/1
  Transpose2/1 -> Zero-Order Hold1/1
  Demux3/1 -> Mux5/3
  euler rate2/1(j) -> MATLAB Function4/1(j)
  Function Caller/8 -> Mux2/8
  In3/1 -> Mux4/1
  MATLAB Function1/3(wz) -> Simulink Function/3(Input2)
  euler rate1/1(j) -> Simulink Function/10(Input9)
  y1/1 -> Extended Kalman Filter1/1
  In1/1 -> Demux3/1

== system quadrotor_model50/Quadrotor/Dynamics Model ==
  tau : Inport  PortDimensions=3
  f : Inport  Port=2  PortDimensions=3
  Initial Angular Velocity : Constant  Value=w_0
  Initial Linear Velocity : Constant  Value=v_0
  Integrator3 : Integrator  InitialConditionSource=external
  Integrator4 : Integrator  InitialConditionSource=external
  Orientation Dynamics : Subsystem  mask{I=I}
      mask prompts: I "Body Inertia Matrix"
      settings: PortSchema="{\"entries\":[{\"content\":{\"sides\":[{\"content\":{\"connectorIds\":[\"In1\"]},\"type\":\"ConnectorPlacement.EquallySpacedRectSide\",\"uuid\":\"c0bebf24-b4c5-4120-b4bc-e257700e30ac\"},{\"content\":{\"connectorIds\":[\"In2\",\"Out1\"],\"side\":\"RIGHT\"},\"type\":\"ConnectorPlacement.EquallySpacedRectSide\",\"uuid\":\"4f6c7abb-67af-4a33-8fe1-31c16aba2e01\"},{\"content\":{\"connectorIds\":[],\"side\":\"TOP\"},\"type\":\"ConnectorPlacement.EquallySpacedRectSide\",\"uuid\":\"8bb59cb6-0e62-4460-a924-40655b1bfaef\"},{\"content\":{\"connectorIds\":[],\"side\":\"HIDDEN\"},\"type\":\"ConnectorPlacement.EquallySpacedRectSide\",\"uuid\":\"077b0ca6-0b74-4b7e-aec6-ebc5a9681944\"}]},\"type\":\"ConnectorPlacement.EquallySpacedConnector\",\"uuid\":\"b5fc50ba-032b-41ac-a5ea-9388df4800bf\"}],\"packageUris\":[\"http://schema.mathworks.com/mf0/Connector/R2020b\"],\"version\":\"1.0\"}"
      mask DialogControl Container3 Prompt: Physical Parameter
      mask Display: disp('Orientation Dynamics')
  Position Dynamics : Subsystem  mask{m=m}
      mask prompts: m "Mass"
      mask DialogControl Container3 Prompt: Physical Parameter
      mask Display: disp('Position Dynamics')
  w : Outport
  v : Outport  Port=2
  a : Outport  Port=3
  wires:
  tau/1 -> Orientation Dynamics/1(tau)
  Integrator3/1 -> Orientation Dynamics/2(w), w/1  "w"
  Position Dynamics/1(dv) -> a/1, Integrator4/1
  Initial Linear Velocity/1 -> Integrator4/2
  Orientation Dynamics/1(dw) -> Integrator3/1
  Integrator4/1 -> v/1  "v"
  f/1 -> Position Dynamics/1(f)
  Initial Angular Velocity/1 -> Integrator3/2

== system quadrotor_model50/Quadrotor/KInematics Model  ==
  w : Inport
  v : Inport  Port=2
  Initial Orientation : Constant  Value=q_0
  Initial Position : Constant  Value=p_0
  Integrator1 : Integrator  InitialConditionSource=external
  Integrator2 : Integrator  InitialConditionSource=external
  Orientation Kinematics : Subsystem
      settings: PortSchema="{\"entries\":[{\"content\":{\"sides\":[{\"content\":{\"connectorIds\":[\"In1\"]},\"type\":\"ConnectorPlacement.EquallySpacedRectSide\",\"uuid\":\"c0bebf24-b4c5-4120-b4bc-e257700e30ac\"},{\"content\":{\"connectorIds\":[\"In2\",\"Out1\"],\"side\":\"RIGHT\"},\"type\":\"ConnectorPlacement.EquallySpacedRectSide\",\"uuid\":\"4f6c7abb-67af-4a33-8fe1-31c16aba2e01\"},{\"content\":{\"connectorIds\":[],\"side\":\"TOP\"},\"type\":\"ConnectorPlacement.EquallySpacedRectSide\",\"uuid\":\"8bb59cb6-0e62-4460-a924-40655b1bfaef\"},{\"content\":{\"connectorIds\":[],\"side\":\"HIDDEN\"},\"type\":\"ConnectorPlacement.EquallySpacedRectSide\",\"uuid\":\"077b0ca6-0b74-4b7e-aec6-ebc5a9681944\"}]},\"type\":\"ConnectorPlacement.EquallySpacedConnector\",\"uuid\":\"b5fc50ba-032b-41ac-a5ea-9388df4800bf\"}],\"packageUris\":[\"http://schema.mathworks.com/mf0/Connector/R2020b\"],\"version\":\"1.0\"}"
  Position Kinematics : Subsystem
  Vector Normalization : Subsystem
      mask Display: disp('v''=v/|v|')
  q : Outport
  p : Outport  Port=2
  wires:
  Position Kinematics/1(dp) -> Integrator2/1
  Orientation Kinematics/1(dq) -> Integrator1/1
  Integrator1/1 -> Vector Normalization/1(v)
  Integrator2/1 -> p/1  "p"
  Initial Position/1 -> Integrator2/2
  Initial Orientation/1 -> Integrator1/2
  w/1 -> Orientation Kinematics/1(w)
  Vector Normalization/1(v') -> Orientation Kinematics/2(q), q/1  "q"
  v/1 -> Position Kinematics/1(v)

== system quadrotor_model50/Quadrotor/quat2Rotm ==
  q : Inport
  Constant : Constant  Value=eye(3)
  Demux : Demux
  Mux : Mux  Inputs=3
  Product1 : Product
  Product2 : Product
  Product3 : Product  Multiplication=Matrix(*)
  Product4 : Product  Multiplication=Matrix(*)
  Skew Operator : Subsystem  Description=S(v)
      mask Display: disp('S(v)')
  Sum : Sum  Inputs=++|
  Sum1 : Sum  Inputs=|++
  Transpose : Math  Operator=transpose  SaturateOnIntegerOverflow=on
  R : Outport
  wires:
  q/1 -> Demux/1  "q"
  Sum1/1 -> R/1  "R"
  Mux/1 -> Transpose/1, Product3/1, Skew Operator/1(v)  "q_v"
  Sum/1 -> Product4/1, Product4/2
  Demux/1 -> Product2/2, Product2/1  "q_0"
  Transpose/1 -> Product3/2
  Demux/2 -> Mux/1
  Demux/3 -> Mux/2
  Demux/4 -> Mux/3
  Product4/1 -> Sum1/1
  Constant/1 -> Product1/2
  Product2/1 -> Product1/1
  Skew Operator/1(S) -> Sum/2
  Product1/1 -> Sum/1
  Product3/1 -> Sum1/2

== system quadrotor_model50/Quadrotor/quat2Rotm2 ==
  q : Inport
  Demux : Demux
  Identity Matrix : dspmtrx3/Identity Matrix  Inherit=off  N=3  Ts=1  dataType=double  isSigned=on  wordLen=16  udDataType=sfix(16)  fracBitsMode=Best precision  numFracBits=15  OutDataTypeStr=double  LastOutDataTypeStr=double
  MATLAB Function : MATLAB Function  TreatAsAtomicUnit=on
  MatrixMultiply : Product  Multiplication=Matrix(*)
  MatrixMultiply1 : Product  Multiplication=Matrix(*)
  Mux : Mux  Inputs=3
  Product : Product
  Product1 : Product
  Sum : Sum  Inputs=++|
  Sum1 : Sum  Inputs=|++
  Transpose : Math  Operator=transpose  SaturateOnIntegerOverflow=on
  R : Outport
  wires:
  q/1 -> Demux/1  "q"
  Mux/1 -> Transpose/1, MatrixMultiply/1, MATLAB Function/1(u)  "q_v"
  Demux/1 -> Product1/2, Product1/1  "q_0"
  Demux/2 -> Mux/1
  Demux/3 -> Mux/2
  Demux/4 -> Mux/3
  Identity Matrix/1 -> Product/2
  Product/1 -> Sum1/1
  MATLAB Function/1(y) -> Sum1/2
  Transpose/1 -> MatrixMultiply/2
  MatrixMultiply/1 -> Sum/2
  Sum/1 -> R/1
  Sum1/1 -> MatrixMultiply1/2, MatrixMultiply1/1
  MatrixMultiply1/1 -> Sum/1
  Product1/1 -> Product/1

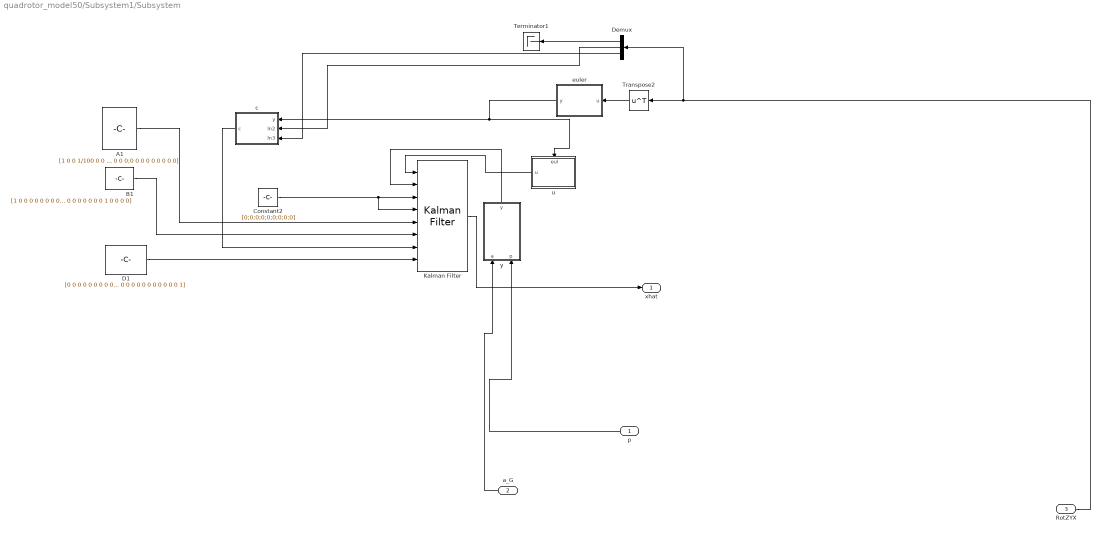
== system quadrotor_model50/Subsystem1/Subsystem ==
  p : Inport
  a_G : Inport  Port=2
  RotZYX : Inport  Port=3
  A1 : Constant  Value=[1 0 0 1/100 0 0 0 0 0;0 1 0 0 1/100 0 0 0 0;0 0 1 0 0 1/100 0 0 0;0 0 0 1 0 0 0 0 0;0 0 0 0 1 0 0 0 0;0 0 0 0 0 1 0 0 0;0 0 0 0 0 0 0 0 0;0 0 0 0 0 0 0 0 0;0 0 0 0 0 0 0 0 0]  SampleTime=1/100
  B1 : Constant  Value=[1 0 0 0 0 0 0 0 0 0 0 0 0;0 1 0 0 0 0 0 0 0 0 0 0 0;0 0 1 0 0 0 0 0 0 0 0 0 0;0 0 0 1 0 0 0 0 0 0 0 0 0;0 0 0 0 1 0 0 0 0 0 0 0 0;0 0 0 0 0 1 0 0 0 0 0 0 0;0 0 0 0 0 0 1 0 0 0 0 0 0;0 0 0 0 0 0 0 1 0 0 0 0 0;0 0 0 0 0 0 0 0 1 0 0 0 0]  SampleTime=1/100
  Constant2 : Constant  Value=[0;0;0;0;0;0;0;0;0]
  D1 : Constant  Value=[0 0 0 0 0 0 0 0 0 1 0 0 0;0 0 0 0 0 0 0 0 0 0 1 0 0;0 0 0 0 0 0 0 0 0 0 0 1 0;0 0 0 0 0 0 0 0 0 0 0 0 1]  SampleTime=1/100
  Demux : Demux  Outputs=3
  Kalman Filter : ctrlSharedLib/Kalman Filter  TimeDomain=Discrete-Time  UseCurrentEstimator=on  ModelSource=Input port  ModelSourceVariable=ss(0.95,1,1,0,1)  A=0.95  B=1  C=1  D=0  NumberOfStates=9  NumberOfInputs=13  NumberOfOutputs=4  InitialEstimateSource=Input port  X0=0  P0=10  UseK=off  UseGH=on  NumberOfProcessNoiseInputs=1  G=[0;0;1/10000;0;0;1/100;0;0;1]  TimeInvariantG=on  H=[0;0;0;0]  TimeInvariantH=on  Q=0.0898  TimeInvariantQ=on  R=diag([0.1,0.1,0.1,0.0008])  TimeInvariantR=on  N=[0,0,0,0]  TimeInvariantN=on  AddInputPort=on  AddEnablePort=off  OutputEstimatedY=off  OutputP=off  Ts=1/100
  Terminator1 : Terminator
  Transpose2 : Math  Operator=transpose  SaturateOnIntegerOverflow=on
  c : Subsystem
  euler : MATLAB Function  TreatAsAtomicUnit=on
  u : Subsystem
      settings: PortSchema="{\"entries\":[{\"content\":{\"sides\":[{\"content\":{\"connectorIds\":[]},\"type\":\"ConnectorPlacement.EquallySpacedRectSide\",\"uuid\":\"26540b1e-a89b-4888-9ec4-fd7f7f630feb\"},{\"content\":{\"connectorIds\":[\"Out1\"],\"side\":\"RIGHT\"},\"type\":\"ConnectorPlacement.EquallySpacedRectSide\",\"uuid\":\"c38f773a-f816-4bcf-adbb-33b029198f6a\"},{\"content\":{\"connectorIds\":[\"In1\"],\"side\":\"TOP\"},\"type\":\"ConnectorPlacement.EquallySpacedRectSide\",\"uuid\":\"b3e9f8ed-a140-475e-aa7e-f57dd0c447f1\"}]},\"type\":\"ConnectorPlacement.EquallySpacedConnector\",\"uuid\":\"be05692c-b490-4b4e-9a7a-7a384c24560c\"}],\"packageUris\":[\"http://schema.mathworks.com/mf0/Connector/R2020b\"],\"version\":\"1.0\"}"
  y : Subsystem
  xhat : Outport
  wires:
  Transpose2/1 -> euler/1(u)
  RotZYX/1 -> Demux/1, Transpose2/1
  Constant2/1 -> Kalman Filter/4, Kalman Filter/3
  A1/1 -> Kalman Filter/5
  D1/1 -> Kalman Filter/8
  B1/1 -> Kalman Filter/6
  c/1(c) -> Kalman Filter/7
  euler/1(y) -> c/1(y), u/1(eul)
  Demux/2 -> c/2(In2)
  u/1(u) -> Kalman Filter/1
  Demux/1 -> Terminator1/1
  Kalman Filter/1 -> xhat/1
  y/1(y) -> Kalman Filter/2
  Demux/3 -> c/3(In3)
  p/1 -> y/2(p)
  a_G/1 -> y/1(a)

== system quadrotor_model50/hover control/Attitude Control (Quaternion)1 ==
  note: Quaternion-based Attitude Control
      | Roll-Pitch-Yaw Attitude Control
  q : Inport
  w_e : Inport  Port=2
  q_ref : Inport  Port=3
  Demux : Demux
  Display : Display
  Gain1 : Gain  Gain=K_q  Multiplication=Matrix(K*u)
  Gain2 : Gain  Gain=K_w  Multiplication=Matrix(K*u)
  Mux : Mux  Inputs=3
  Quaternion Conjugate : aerolibutil/Quaternion Conjugate
      settings: SourceProductBaseCode=AE
  Quaternion Multiplication : aerolibutil/Quaternion Multiplication
  Sum : Sum  Inputs=|+-
  Terminator : Terminator
  tau : Outport
  wires:
  w_e/1 -> Gain2/1
  Quaternion Conjugate/1 -> Quaternion Multiplication/2
  Sum/1 -> tau/1
  Mux/1 -> Display/1, Gain1/1
  Gain2/1 -> Sum/2
  Gain1/1 -> Sum/1
  Demux/1 -> Terminator/1
  Demux/3 -> Mux/2
  Demux/4 -> Mux/3
  Demux/2 -> Mux/1
  Quaternion Multiplication/1 -> Demux/1
  q_ref/1 -> Quaternion Multiplication/1
  q/1 -> Quaternion Conjugate/1

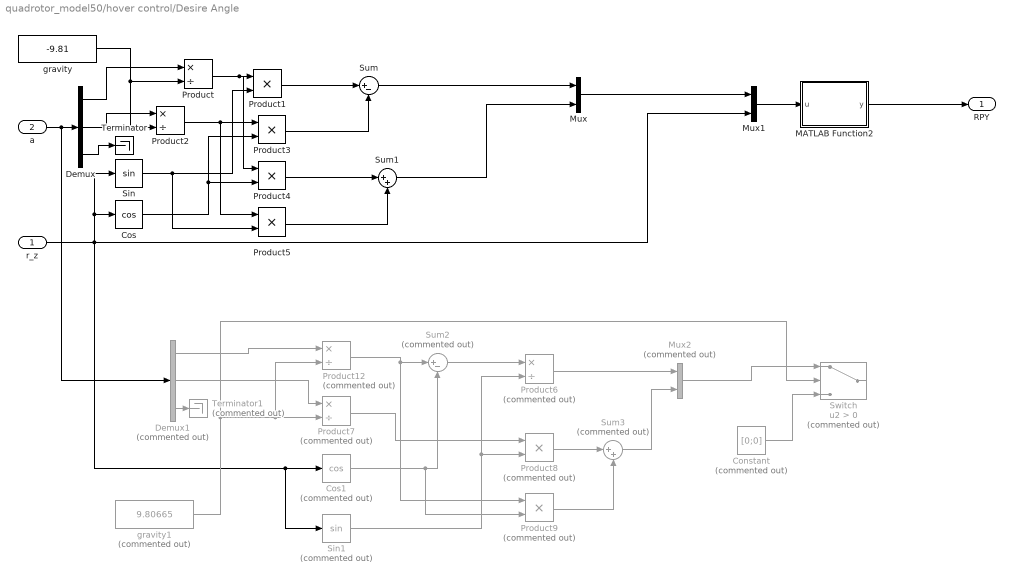
== system quadrotor_model50/hover control/Desire Angle ==
  r_z : Inport
  a : Inport  Port=2
  Constant : Constant  Commented=on  Value=[0;0]
  Cos : Trigonometry  Operator=cos
  Cos1 : Trigonometry  Commented=on  Operator=cos
  Demux : Demux  Outputs=3
  Demux1 : Demux  Commented=on  Outputs=3
  MATLAB Function2 : MATLAB Function  TreatAsAtomicUnit=on
  Mux : Mux  Inputs=2
  Mux1 : Mux  Inputs=2
  Mux2 : Mux  Commented=on  Inputs=2
  Product : Product  Inputs=*/
  Product{1,3..5} (4 alike) : Product
  Product12 : Product  Commented=on  Inputs=*/
  Product2 : Product  Inputs=*/
  Product6 : Product  Commented=on  Inputs=*/
  Product7 : Product  Commented=on  Inputs=*/
  Product8 : Product  Commented=on
  Product9 : Product  Commented=on
  Sin : Trigonometry
  Sin1 : Trigonometry  Commented=on
  Sum : Sum  Inputs=|+-
  Sum1 : Sum  Inputs=|++
  Sum2 : Sum  Commented=on  Inputs=|+-
  Sum3 : Sum  Commented=on  Inputs=|++
  Switch : Switch  Commented=on  Criteria=u2 > Threshold
  Terminator : Terminator
  Terminator1 : Terminator  Commented=on
  gravity : Constant  Value=-9.81  VectorParams1D=off
  gravity1 : Constant  Commented=on  Value=9.80665  VectorParams1D=off
  RPY : Outport
  wires:
  Mux1/1 -> MATLAB Function2/1(u)
  Demux/1 -> Product/1
  gravity/1 -> Product/2, Product2/2
  Product/1 -> Product4/1, Product1/1
  Sin/1 -> Product5/2, Product1/2
  Product1/1 -> Sum/1
  Demux/2 -> Product2/1
  Product2/1 -> Product5/1, Product3/1
  Cos/1 -> Product4/2, Product3/2
  Product3/1 -> Sum/2
  Sum/1 -> Mux/1
  Product4/1 -> Sum1/1
  Product5/1 -> Sum1/2
  Sum1/1 -> Mux/2
  Demux/3 -> Terminator/1
  a/1 -> Demux1/1, Demux/1
  r_z/1 -> Sin1/1, Cos1/1, Mux1/2, Sin/1, Cos/1
  Demux1/1 -> Product12/1
  Product12/1 -> Product9/1, Sum2/1
  Cos1/1 -> Product9/2, Sum2/2
  Sum2/1 -> Product6/1
  Sin1/1 -> Product8/2, Product6/2
  Product6/1 -> Mux2/1
  MATLAB Function2/1(y) -> RPY/1
  Demux1/2 -> Product7/1
  Product7/1 -> Product8/1
  Product8/1 -> Sum3/1
  Product9/1 -> Sum3/2
  Sum3/1 -> Mux2/2
  gravity1/1 -> Switch/2, Product7/2, Product12/2
  Mux2/1 -> Switch/1
  Constant/1 -> Switch/3
  Demux1/3 -> Terminator1/1
  Mux/1 -> Mux1/1

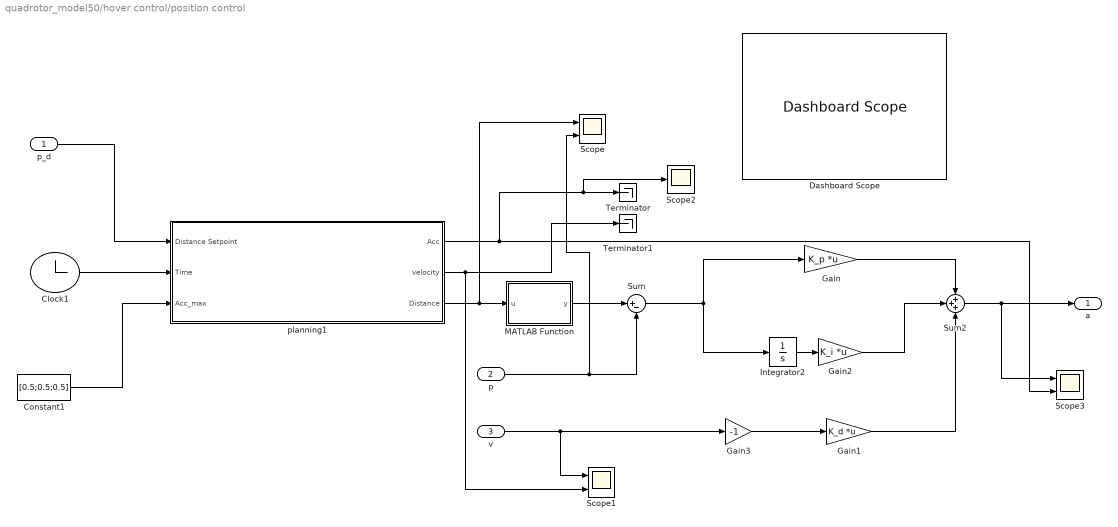
== system quadrotor_model50/hover control/position control ==
  p_d : Inport
  p : Inport  Port=2
  v : Inport  Port=3
  Clock1 : Clock
  Constant1 : Constant  Value=[0.5;0.5;0.5]
  Dashboard Scope : DashboardScope
  Gain : Gain  Gain=K_p  Multiplication=Matrix(K*u)
  Gain1 : Gain  Gain=K_d  Multiplication=Matrix(K*u)
  Gain2 : Gain  Gain=K_i  Multiplication=Matrix(K*u)
  Gain3 : Gain  Gain=-1
  Integrator2 : Integrator
  MATLAB Function : MATLAB Function  TreatAsAtomicUnit=on
  Scope : Scope  NumInputPorts=2
  Scope1 : Scope  NumInputPorts=2
  Scope2 : Scope
  Scope3 : Scope  NumInputPorts=2
  Sum : Sum  Inputs=|+-
  Sum2 : Sum  Inputs=+++
  Terminator : Terminator
  Terminator1 : Terminator
  planning1 : Subsystem
  a : Outport  SampleTime=1/50
  wires:
  Constant1/1 -> planning1/3(Acc_max)
  Sum2/1 -> Scope3/1, a/1
  p/1 -> Scope/2, Sum/2
  planning1/1("Acc ") -> Scope3/2, Scope2/1, Terminator/1
  planning1/2(velocity) -> Scope1/2, Terminator1/1
  Sum/1 -> Gain/1, Integrator2/1
  Gain/1 -> Sum2/1
  v/1 -> Scope1/1, Gain3/1
  Gain3/1 -> Gain1/1
  Gain1/1 -> Sum2/3
  Integrator2/1 -> Gain2/1
  Gain2/1 -> Sum2/2
  p_d/1 -> planning1/1(Distance Setpoint)
  MATLAB Function/1(y) -> Sum/1
  planning1/3(Distance) -> Scope/1, MATLAB Function/1(u)
  Clock1/1 -> planning1/2(Time)
